simulink model "C01_2"  (R2021a)
settings: Solver=VariableStepAuto  StartTime=0.0  StopTime=10.0  RelTol=1e-3
settings Model: Creator=riobe  LastModifiedBy=riobe

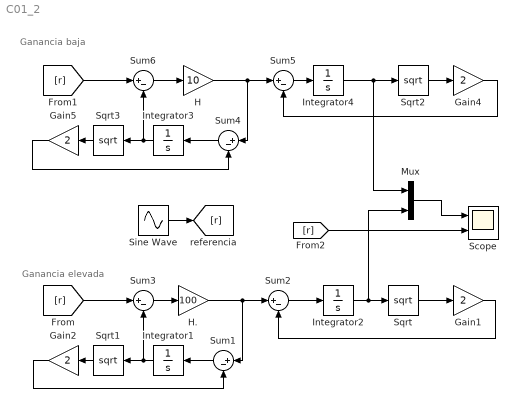
== system C01_2 ==
  note: Ganancia elevada
  note: Ganancia baja
  Gain{1..2,4..5} (4 alike) : Gain  Gain=2
  H : Gain  Gain=10
  H. : Gain  Gain=100
  Integrator{1..4} (4 alike) : Integrator
  Mux : Mux  Inputs=2
  Scope : Scope  NumInputPorts=2
  Sine Wave : Sin  Frequency=2  SampleTime=0
  Sqrt{,1..3} (4 alike) : Sqrt  SaturateOnIntegerOverflow=on
  Sum{1..6} (6 alike) : Sum  Inputs=|+-
  wires:
  Sqrt/1 -> Gain1/1
  Integrator2/1 -> Mux/2, Sqrt/1
  Sum2/1 -> Integrator2/1
  Gain1/1 -> Sum2/2
  Integrator1/1 -> Sqrt1/1, Sum3/2
  Sum1/1 -> Integrator1/1
  Gain2/1 -> Sum1/2
  Sqrt1/1 -> Gain2/1
  H./1 -> Sum1/1, Sum2/1
  Sum3/1 -> H./1
  Integrator4/1 -> Mux/1, Sqrt2/1
  Sum5/1 -> Integrator4/1
  Sqrt2/1 -> Gain4/1
  Sqrt3/1 -> Gain5/1
  Integrator3/1 -> Sqrt3/1, Sum6/2
  Gain4/1 -> Sum5/2
  Gain5/1 -> Sum4/2
  Sum4/1 -> Integrator3/1
  H/1 -> Sum4/1, Sum5/1
  Sum6/1 -> H/1
  Sine Wave/1 -> [r]
  [r] -> Sum3/1
  [r] -> Sum6/1
  [r] -> Scope/2
  Mux/1 -> Scope/1
